simulink model "basicFeedbackSystem"  (R2019b)
settings: Solver=VariableStepAuto  StartTime=0.0  StopTime=10.0  RelTol=1e-3
settings Model: Creator=23731  LastModifiedBy=23731

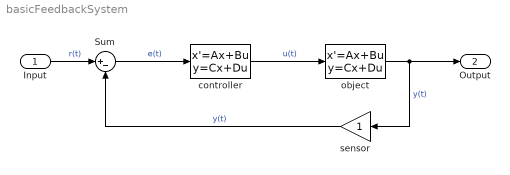
== system basicFeedbackSystem ==
  Input : Inport
  Sum : Sum  Inputs=|+-
  controller : StateSpace  InitialCondition=0
  object : StateSpace  InitialCondition=0
  sensor : Gain
  Output : Outport  Port=2
  wires:
  Sum/1 -> controller/1  "e(t)"
  controller/1 -> object/1  "u(t)"
  sensor/1 -> Sum/2  "y(t)"
  object/1 -> Output/1, sensor/1  "y(t)"
  Input/1 -> Sum/1  "r(t)"
